simulink model "realim_estados_i"  (R2026a)
settings: Solver=ode4  StopTime=10  FixedStep=1e-3
values from neighbouring files (symbols this model uses):
  A = [0,         1,      0,      0 ... (first row only)    [realim_estados_i.m]
  B = [       0 ... (first row only)    [realim_estados_i.m]
  C = [1,         0,      0,      0 ... (first row only)    [realim_estados_i.m]
  C_new = [0, 0, 1, 0]    [realim_estados_i.m]
  D = [0 ... (first row only)    [realim_estados_i.m]
  K_ext = place(Aext, Bext, [z1_k, z2_k, z3_k, z4_k, z5_k])    [realim_estados_i.m]
  L_d = place(Ad2', Cd2', [l1_z, l2_z, l3_z, l4_z])'    [realim_estados_i.m]
  Ts = 20e-3    (= 0.02)    [graficador_final.m]    (also in graficador_promedios.m; realim_estados_i.m; test_graficos.m; untitled4.m)
undefined symbols (not defined in the file or in its folder): Ad2, Bd2, Cd2
settings Model: Creator=Dante P  LastModifiedBy=Dante P

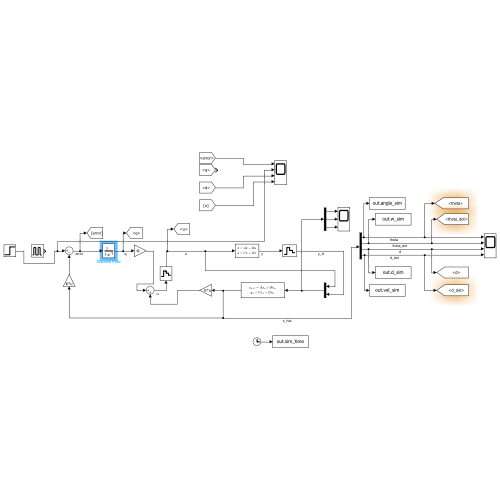
[thumbnail: Simulink's stored preview of the top-level diagram]
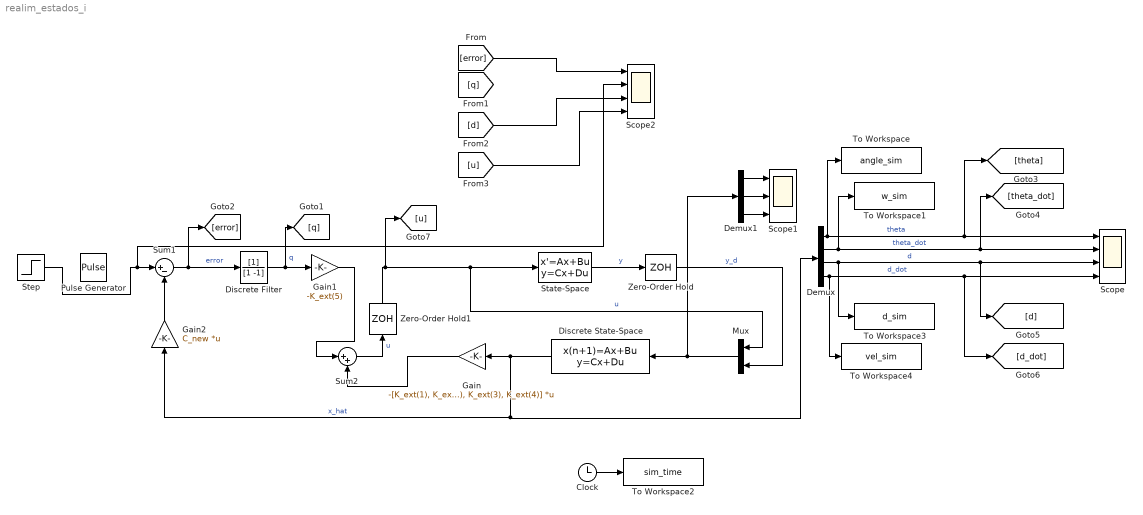
== system realim_estados_i ==
  Clock : Clock
  Demux : Demux
  Demux1 : Demux  Outputs=3
  Discrete Filter : DiscreteFilter  Denominator=[1 -1]
  Discrete State-Space : DiscreteStateSpace  A=Ad2 - L_d * Cd2  B=[Bd2, L_d]  C=eye(4)  D=zeros(4,3)  SampleTime=Ts
  Gain : Gain  Gain=-[K_ext(1), K_ext(2), K_ext(3), K_ext(4)]  Multiplication=Matrix(K*u)
  Gain1 : Gain  Gain=-K_ext(5)
  Gain2 : Gain  Gain=C_new  Multiplication=Matrix(K*u)
  Mux : Mux  Inputs=2
  Pulse Generator : DiscretePulseGenerator  PulseType=Time based  Amplitude=15  Period=20  PulseWidth=50
  Scope : Scope  NumInputPorts=4
      settings: ActiveDisplayYMinimum=-0.021316062002409882  ActiveDisplayYMaximum=0.1018530201492205
  Scope1 : Scope  NumInputPorts=3
      settings: ActiveDisplayYMinimum=-6.8750627406225915  ActiveDisplayYMaximum=6.8750627406225915
  Scope2 : Scope  NumInputPorts=4
      settings: ActiveDisplayYMinimum=-1.2499999999999998  ActiveDisplayYMaximum=11.25  DataLoggingVariableName=ScopeData2
  State-Space : StateSpace  A=A  B=B  C=C  D=D  InitialCondition=0
  Step : Step  FinalValue=10  SampleTime=Ts
  Sum1 : Sum  Inputs=|+-
  Sum2 : Sum  Inputs=|++
  To Workspace : ToWorkspace  VariableName=angle_sim  SampleTime=-1
  To Workspace1 : ToWorkspace  VariableName=w_sim  SampleTime=-1
  To Workspace2 : ToWorkspace  VariableName=sim_time  SampleTime=0.02
  To Workspace3 : ToWorkspace  VariableName=d_sim  SampleTime=-1
  To Workspace4 : ToWorkspace  VariableName=vel_sim  SampleTime=-1
  Zero-Order Hold : ZeroOrderHold  SampleTime=Ts
  Zero-Order Hold1 : ZeroOrderHold  SampleTime=Ts
  wires:
  Gain/1 -> Sum2/2
  Clock/1 -> To Workspace2/1
  Discrete State-Space/1 -> Gain2/1, Demux/1, Gain/1  "x_hat"
  Zero-Order Hold/1 -> Mux/2  "y_d"
  Mux/1 -> Demux1/1, Discrete State-Space/1
  Demux/1 -> To Workspace/1, [theta], Scope/1  "theta"
  Demux/2 -> To Workspace1/1, [theta_dot], Scope/2  "theta_dot"
  Demux/4 -> To Workspace4/1, [d_dot], Scope/4  "d_dot"
  Demux/3 -> To Workspace3/1, [d], Scope/3  "d"
  Zero-Order Hold1/1 -> [u], Mux/1, State-Space/1  "u"
  Demux1/2 -> Scope1/2
  Demux1/1 -> Scope1/1
  State-Space/1 -> Zero-Order Hold/1  "y"
  Demux1/3 -> Scope1/3
  Discrete Filter/1 -> [q], Gain1/1  "q"
  Gain1/1 -> Sum2/1
  Sum1/1 -> Discrete Filter/1, [error]  "error"
  Step/1 -> Scope2/2, Sum1/1
  Sum2/1 -> Zero-Order Hold1/1  "u"
  [error] -> Scope2/1
  [u] -> Scope2/4
  [d] -> Scope2/3
  Gain2/1 -> Sum1/2
